simulink library "ESTS_LSM_SM"  (R2023b)
settings: Solver=VariableStepAuto  StartTime=0.0  StopTime=10.0  RelTol=1e-3
undefined symbols (not defined in the file): p_CrnrgStfnFr_Nprad, p_CrnrgStfnRe_Nprad
libraries: VUT_lib x1
settings Model: Creator=blatak  LastModifiedBy=blatak

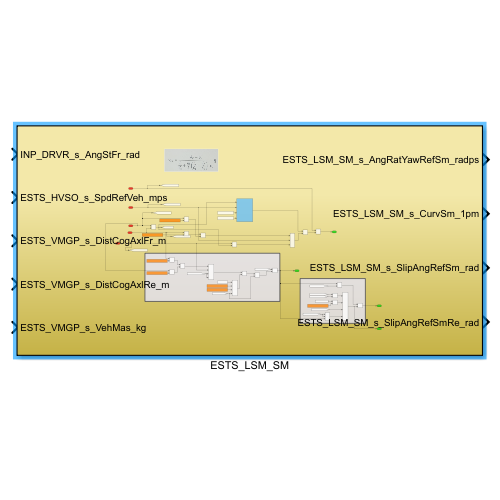
[thumbnail: Simulink's stored preview of the top-level diagram]
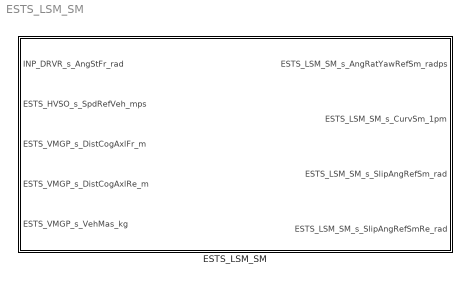
== system ESTS_LSM_SM ==
  ESTS_LSM_SM : Subsystem

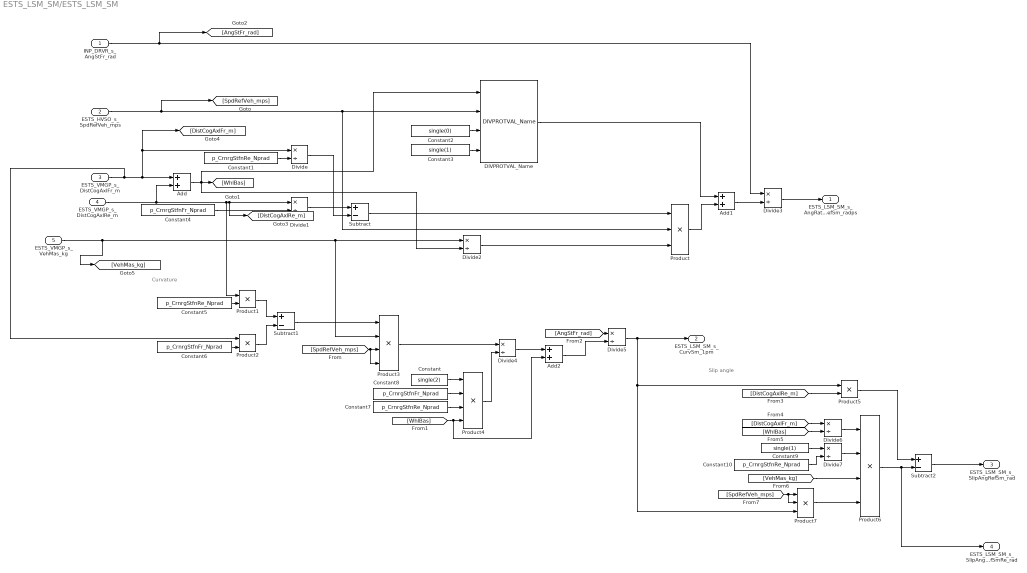
== system ESTS_LSM_SM/ESTS_LSM_SM ==
  note: Curvature
  note: Slip angle
  INP_DRVR_s_AngStFr_rad : Inport  Description=|
      | Steering wheel angle front - calculated as an average FL and FR,
      | used for single track model, later more sophisticated calculation method needed 
      | than only an average
  ESTS_HVSO_s_SpdRefVeh_mps : Inport  Description=Estimated reference vehicle speed  Port=2
  ESTS_VMGP_s_DistCogAxlFr_m : Inport  Description=X distance from front axle (wheel center) to cog  Port=3
  ESTS_VMGP_s_DistCogAxlRe_m : Inport  Description=X distance from rear axle (wheel center) to cog  Port=4
  ESTS_VMGP_s_VehMas_kg : Inport  Description=Vehicle mass  Port=5
  Add : Sum
  Add1 : Sum
  Add2 : Sum
  Constant : Constant  Value=single(2)
  Constant1 : Constant  Description=Parameter - rear axle cornering stiffness  Value=p_CrnrgStfnRe_Nprad
  Constant10 : Constant  Value=p_CrnrgStfnRe_Nprad
  Constant2 : Constant  Value=single(0)
  Constant3 : Constant  Value=single(1)
  Constant4 : Constant  Description=Parameter - front axle cornering stiffness  Value=p_CrnrgStfnFr_Nprad
  Constant5 : Constant  Value=p_CrnrgStfnRe_Nprad
  Constant6 : Constant  Value=p_CrnrgStfnFr_Nprad
  Constant7 : Constant  Value=p_CrnrgStfnRe_Nprad
  Constant8 : Constant  Value=p_CrnrgStfnFr_Nprad
  Constant9 : Constant  Value=single(1)
  DIVPROTVAL_Name : VUT_lib/DIVPROTVAL_Name  SystemSampleTime=-1  VariantActivationTime=update diagram  AllowFlexibleInterface=on  Latency=0  AutoFrameSizeCalculation=off
  Divide{,1..3} (4 alike) : Product  Inputs=*/  RndMeth=Zero  SaturateOnIntegerOverflow=on
  Divide{4..7} (4 alike) : Product  Inputs=*/
  Product : Product  Inputs=3
  Product1 : Product
  Product2 : Product
  Product3 : Product  Inputs=4
  Product4 : Product  Inputs=4
  Product5 : Product
  Product6 : Product  Inputs=4
  Product7 : Product  Inputs=3
  Subtract : Sum  Inputs=+-
  Subtract1 : Sum  Inputs=+-
  Subtract2 : Sum  Inputs=+-
  ESTS_LSM_SM_s_AngRatYawRefSm_radps : Outport  Description=Reference yaw velocity from steday state model (formula)
  ESTS_LSM_SM_s_CurvSm_1pm : Outport  Description=Curvature from steady state (single track) model (formula)  Port=2
  ESTS_LSM_SM_s_SlipAngRefSm_rad : Outport  Description=Reference slip angle in cog from steady state model (formula)  Port=3
  ESTS_LSM_SM_s_SlipAngRefSmRe_rad : Outport  Description=Reference slip angle on rear axle from steady state model (formula)  Port=4
  wires:
  Constant2/1 -> DIVPROTVAL_Name/3
  Add2/1 -> Divide5/2
  [SpdRefVeh_mps] -> Product7/2, Product7/1
  ESTS_HVSO_s_SpdRefVeh_mps/1 -> DIVPROTVAL_Name/2, Product/2, [SpdRefVeh_mps]
  [SpdRefVeh_mps] -> Product3/4, Product3/3
  Constant10/1 -> Divide7/2
  [WhlBas] -> Divide6/2
  Divide7/1 -> Product6/2
  Add1/1 -> Divide3/2
  [DistCogAxlFr_m] -> Divide6/1
  Product1/1 -> Subtract1/1
  ESTS_VMGP_s_DistCogAxlFr_m/1 -> [DistCogAxlFr_m], Divide/1, Add/1, Product2/1
  Product2/1 -> Subtract1/2
  Product5/1 -> Subtract2/1
  Add/1 -> [WhlBas], Divide2/2, DIVPROTVAL_Name/1
  Constant8/1 -> Product4/2
  ESTS_VMGP_s_VehMas_kg/1 -> Product3/2, Divide2/1, [VehMas_kg]
  Product/1 -> Add1/2
  Constant/1 -> Product4/1
  Product3/1 -> Divide4/1
  [DistCogAxlRe_m] -> Product5/2
  ESTS_VMGP_s_DistCogAxlRe_m/1 -> [DistCogAxlRe_m], Divide1/1, Product1/1, Add/2
  INP_DRVR_s_AngStFr_rad/1 -> [AngStFr_rad], Divide3/1
  Divide2/1 -> Product/3
  Product7/1 -> Product6/4
  [WhlBas] -> Add2/2, Product4/4
  Product4/1 -> Divide4/2
  [AngStFr_rad] -> Divide5/1
  Subtract2/1 -> ESTS_LSM_SM_s_SlipAngRefSm_rad/1
  Divide6/1 -> Product6/1
  Divide5/1 -> ESTS_LSM_SM_s_CurvSm_1pm/1, Product7/3, Product5/1
  Constant4/1 -> Divide1/2
  Constant5/1 -> Product1/2
  DIVPROTVAL_Name/1 -> Add1/1
  Divide4/1 -> Add2/1
  Divide/1 -> Subtract/2
  [VehMas_kg] -> Product6/3
  Divide3/1 -> ESTS_LSM_SM_s_AngRatYawRefSm_radps/1
  Constant9/1 -> Divide7/1
  Subtract1/1 -> Product3/1
  Constant6/1 -> Product2/2
  Constant7/1 -> Product4/3
  Constant1/1 -> Divide/2
  Product6/1 -> ESTS_LSM_SM_s_SlipAngRefSmRe_rad/1, Subtract2/2
  Constant3/1 -> DIVPROTVAL_Name/4
  Divide1/1 -> Subtract/1
  Subtract/1 -> Product/1
